simulink model "ExoTeR"  (R2019b)
settings: Solver=VariableStepAuto  StartTime=0.0  StopTime=t(end)  MaxStep=0.001  RelTol=1e-6  AbsTol=1e-6  EnableMultiTasking=on
undefined symbols (not defined in the file): a2, a3, d1, d4, d5, d6, g, Housing, ki, kp, l, m1, m2, m3, m4, m5, mu, q, rollef, s, slope, theta, vehicleMass, wheelMass, wheelRadius, x, X, xef, Y, yef, Z, zGC
libraries: sm_lib x187, fl_lib x99, nesl_utility x45, ee_lib x12, simulink x6
(part 6 of 7)

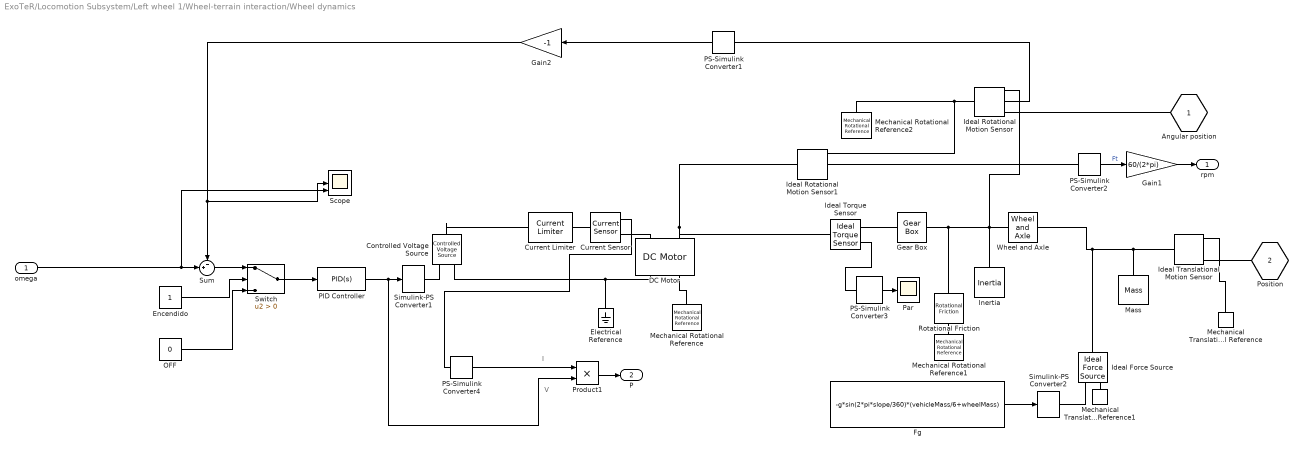
== system ExoTeR/Locomotion Subsystem/Left wheel 1/Wheel-terrain interaction/Wheel dynamics ==
  note: V
  note: I
  omega : Inport
  Controlled Voltage Source : fl_lib/Electrical/Electrical Sources/Controlled Voltage Source
  Current Limiter : ee_lib/Semiconductors & Converters/Current Limiter  iLim=0.5 A  vLim=0.01 V  gLim=1e-3 1/Ohm  thermal_mass=100 J/K  initial_temperature=298.15 K
      settings: SourceProductName=Simscape Electrical  SourceProductBaseCode=PS  InternalSimscapePortConfiguration="{\"Bottom\":[],\"Left\":[{\"id\":\"p\",\"label\":\"+\",\"type\":\"foundation.electrical.electrical\"}],\"Right\":[{\"id\":\"n\",\"label\":\"-\",\"type\":\"foundation.electrical.electrical\"}],\"Top\":[]}"
  Current Sensor : fl_lib/Electrical/Electrical Sensors/Current Sensor
  DC Motor : ee_lib/Electromechanical/Brushed Motors/DC Motor  parameterization=2  Ra=3.9 Ohm  La=0.000363 H  emf_or_torque=2  Kv=0.0011 V/rpm  Ki=10.9 mN*m/A  T_stall=0.0237 N*m  w_max=10200 rpm  w_rated=1.5e+4 rpm  P_rated=0.08 W  V_rated=12 V  J=4.36 g*cm^2  lam_param=2  lam=Bm N*m/(rad/s)  i_noload=0.0458 A  V_i_noload=11.657 V  speed0=0 rpm  alpha=3.93e-3 1/K  Tmeas=25 degC  thermal_mass=100 J/K  initial_temperature=25 degC
      settings: SourceProductName=Simscape Electrical
  Electrical Reference : fl_lib/Electrical/Electrical Elements/Electrical Reference
  Encendido : Constant
  Fg : Constant  Value=-g*sin(2*pi*slope/360)*(vehicleMass/6+wheelMass)
  Gain1 : Gain  Gain=60/(2*pi)
  Gain2 : Gain  Gain=-1
  Gear Box : fl_lib/Mechanical/Mechanisms/Gear Box  ratio=675.545  t_in_specify=off  t_in_priority=None  t_in=0 N*m  t_in_nominal_specify=off  t_in_nominal_unit=N*m  t_in_nominal_value=1  t_out_specify=off  t_out_priority=None  t_out=0 N*m  t_out_nominal_specify=off  t_out_nominal_unit=N*m  t_out_nominal_value=1
  Ideal Force Source : fl_lib/Mechanical/Mechanical Sources/Ideal Force Source
  Ideal Rotational Motion Sensor : fl_lib/Mechanical/Mechanical Sensors/Ideal Rotational Motion Sensor  offset=0 rad
  Ideal Rotational Motion Sensor1 : fl_lib/Mechanical/Mechanical Sensors/Ideal Rotational Motion Sensor  offset=0 rad
  Ideal Torque Sensor : fl_lib/Mechanical/Mechanical Sensors/Ideal Torque Sensor
  Ideal Translational Motion Sensor : fl_lib/Mechanical/Mechanical Sensors/Ideal Translational Motion Sensor  offset=0 m
  Inertia : fl_lib/Mechanical/Rotational Elements/Inertia  inertia=Jw kg*m^2  w_specify=off  w_priority=None  w=0 rad/s  w_nominal_specify=off  w_nominal_unit=rad/s  w_nominal_value=1  t_specify=off  t_priority=None  t=0 N*m  t_nominal_specify=off  t_nominal_unit=N*m  t_nominal_value=1
  Mass : fl_lib/Mechanical/Translational Elements/Mass  mass=vehicleMass/6+wheelMass kg  v_specify=off  v_priority=None  v=0 m/s  v_nominal_specify=off  v_nominal_unit=m/s  v_nominal_value=1  f_specify=off  f_priority=None  f=0 N  f_nominal_specify=off  f_nominal_unit=N  f_nominal_value=1
  Mechanical Rotational Reference : fl_lib/Mechanical/Rotational Elements/Mechanical Rotational Reference
  Mechanical Rotational Reference1 : fl_lib/Mechanical/Rotational Elements/Mechanical Rotational Reference
  Mechanical Rotational Reference2 : fl_lib/Mechanical/Rotational Elements/Mechanical Rotational Reference
  Mechanical Translational Reference : fl_lib/Mechanical/Translational Elements/Mechanical Translational Reference
  Mechanical Translational Reference1 : fl_lib/Mechanical/Translational Elements/Mechanical Translational Reference
  OFF : Constant  Value=0
  PID Controller : simulink/Continuous/PID Controller  Controller=PID  Form=Parallel  TimeDomain=Continuous-time  SampleTime=-1  IntegratorMethod=Forward Euler  FilterMethod=Forward Euler  ControllerParametersSource=internal  P=kp  I=ki  D=0  UseFilter=on  N=100  TunerSelectOption=Transfer Function Based (PID Tuner App)  InitialConditionSource=internal  InitialConditionForIntegrator=0  InitialConditionForFilter=0  DifferentiatorICPrevScaledInput=0  ExternalReset=none  TrackingMode=off  Kt=1  LimitOutput=on  UpperSaturationLimit=12  LowerSaturationLimit=-12  LinearizeAsGain=on  AntiWindupMode=back-calculation  Kb=1  POutMin=[]  POutMax=[]  IOutMin=[]  IOutMax=[]  DOutMin=[]  DOutMax=[]  NOutMin=[]  NOutMax=[]  SumOutMin=[]  SumOutMax=[]  SaturationOutMin=[]  SaturationOutMax=[]  PParamMin=[]  PParamMax=[]  IParamMin=[]  IParamMax=[]  DParamMin=[]  DParamMax=[]  NParamMin=[]  NParamMax=[]  KbParamMin=[]  KbParamMax=[]  KtParamMin=[]  KtParamMax=[]  KbOutMin=[]  KbOutMax=[]  KtOutMin=[]  KtOutMax=[]  IntegratorOutMin=[]  IntegratorOutMax=[]  FilterOutMin=[]  FilterOutMax=[]  SumI1OutMin=[]  SumI1OutMax=[]  SumI2OutMin=[]  SumI2OutMax=[]  SumI3OutMin=[]  SumI3OutMax=[]  SumI4OutMin=[]  SumI4OutMax=[]  SumDOutMin=[]  SumDOutMax=[]  DifferentiatorOutMin=[]  DifferentiatorOutMax=[]  FilterDiffOutCoefMin=[]  FilterDiffOutCoefMax=[]  ReciprocalOutMin=[]  ReciprocalOutMax=[]  SumDenOutMin=[]  SumDenOutMax=[]  SumNumOutMin=[]  SumNumOutMax=[]  DivideOutMin=[]  DivideOutMax=[]  IntegratorContinuousStateAttributes=''  IntegratorStateMustResolveToSignalObject=off  IntegratorRTWStateStorageClass=Auto  FilterContinuousStateAttributes=''  FilterStateMustResolveToSignalObject=off  FilterRTWStateStorageClass=Auto  ParallelPVariant=InternalParameters  IdealPVariant=Disabled  IVariant=InternalParameters  DVariant=InternalParameters  IntegratorVariant=Continuous  SatVariant=Enabled  AWVariant=BackCalculation  PCopyVariant=Disabled  TRVariant=Disabled  FdbkBlocksVariant=Forward  IdealPFdbkVariant=Disabled  SatFdbkVariant=Disabled  DerivativeFilterVariant=ContFilter  NVariant=InternalParameters  NCopyVariant=Disabled  FilterICVariant=InternalICsFilter  IntegratorICVariant=InternalICs  ExternalResetVariant=Disabled  TRSumVariant=Passthrough  SumFdbkVariant=Disabled  SumVariant=Sum_PID
  PS-Simulink Converter{1..4} (4 alike) : nesl_utility/PS-Simulink Converter  PhysicalDomain=network_engine_domain  SubClassName=ps_output  LeftPortType=input  RightPortType=output  PseudoPeriodic=off  Frequencies=[]  Unit=1  AffineConversion=off
  Par : Scope
  Product1 : Product
  Rotational Friction : fl_lib/Mechanical/Rotational Elements/Rotational Friction  brkwy_trq=(vehicleMass/6+wheelMass)*g*cos(2*pi*slope/360)*mu*wheelRadius*s + (vehicleMass/6+wheelMass)*g*cos(2*pi*slope/360)*mu*0.1*wheelRadius*(1-s) N*m  brkwy_vel=0.060623 rad/s  Col_trq=((vehicleMass/6+wheelMass)*g*cos(2*pi*slope/360)*mu*wheelRadius*s + (vehicleMass/6+wheelMass)*g*cos(2*pi*slope/360)*mu*0.1*wheelRadius*(1-s))*0.9 N*m  visc_coef=0.001 N*m/(rad/s)  w_specify=off  w_priority=None  w=0 rad/s  w_nominal_specify=off  w_nominal_unit=rad/s  w_nominal_value=1  t_specify=off  t_priority=None  t=0 N*m  t_nominal_specify=off  t_nominal_unit=N*m  t_nominal_value=1
      settings: SourceProductName=Simscape
  Scope : Scope  NumInputPorts=3
  Simulink-PS Converter1 : nesl_utility/Simulink-PS Converter  PhysicalDomain=network_engine_domain  SubClassName=ps_input  LeftPortType=input  RightPortType=output  PseudoPeriodic=off  Frequencies=[]  NoiseDistribution=none  NoiseParameters=[]  Unit=1  AffineConversion=off  FilteringAndDerivatives=zero  SimscapeFilterOrder=1  InputFilterTimeConstant=0.001  UdotUserProvided=1
  Simulink-PS Converter2 : nesl_utility/Simulink-PS Converter  PhysicalDomain=network_engine_domain  SubClassName=ps_input  LeftPortType=input  RightPortType=output  PseudoPeriodic=off  Frequencies=[]  NoiseDistribution=none  NoiseParameters=[]  Unit=1  AffineConversion=off  FilteringAndDerivatives=zero  SimscapeFilterOrder=1  InputFilterTimeConstant=0.001  UdotUserProvided=1
  Sum : Sum  Inputs=-+|
  Switch : Switch  Criteria=u2 > Threshold
  Wheel and Axle : fl_lib/Mechanical/Mechanisms/Wheel and Axle  R=wheelRadius m  or=1  t_specify=off  t_priority=None  t=0 N*m  t_nominal_specify=off  t_nominal_unit=N*m  t_nominal_value=1  f_specify=off  f_priority=None  f=0 N  f_nominal_specify=off  f_nominal_unit=N  f_nominal_value=1
      settings: SourceProductName=Simscape
  Angular position : PMIOPort  Side=Right
  Position : PMIOPort  Port=2  Side=Right
  rpm : Outport
  P : Outport  Port=2
  wires:
  PS-Simulink Converter2/1 -> Gain1/1  "Ft"
  Gain1/1 -> rpm/1
  Fg/1 -> Simulink-PS Converter2/1
  PID Controller/1 -> Product1/2, Simulink-PS Converter1/1
  PS-Simulink Converter1/1 -> Gain2/1
  omega/1 -> Scope/3, Sum/2
  Gain2/1 -> Scope/2, Sum/1
  Encendido/1 -> Switch/2
  OFF/1 -> Switch/3
  Switch/1 -> PID Controller/1
  Sum/1 -> Switch/1
  PS-Simulink Converter3/1 -> Par/1
  PS-Simulink Converter4/1 -> Product1/1
  Product1/1 -> P/1
  connections:
  Inertia/LConn1 -- Rotational Friction/LConn1 -- Gear Box/RConn1 -- Ideal Rotational Motion Sensor/RConn1 -- Wheel and Axle/LConn1
  DC Motor/RConn2 -- Mechanical Rotational Reference/LConn1
  Ideal Rotational Motion Sensor1/LConn1 -- Ideal Torque Sensor/LConn1 -- DC Motor/LConn2
  Mechanical Translational Reference/LConn1 -- Ideal Translational Motion Sensor/RConn1
  Electrical Reference/LConn1 -- DC Motor/RConn1 -- Controlled Voltage Source/RConn2
  Simulink-PS Converter1/RConn1 -- Controlled Voltage Source/RConn1
  Mechanical Rotational Reference1/LConn1 -- Rotational Friction/RConn1
  Ideal Rotational Motion Sensor/RConn3 -- Angular position/RConn1
  Ideal Translational Motion Sensor/RConn3 -- Position/RConn1
  Mechanical Rotational Reference2/LConn1 -- Ideal Rotational Motion Sensor1/RConn1 -- Ideal Rotational Motion Sensor/LConn1
  Ideal Rotational Motion Sensor1/RConn2 -- PS-Simulink Converter2/LConn1
  Simulink-PS Converter2/RConn1 -- Ideal Force Source/RConn1
  Mechanical Translational Reference1/LConn1 -- Ideal Force Source/RConn2
  Ideal Translational Motion Sensor/LConn1 -- Wheel and Axle/RConn1 -- Ideal Force Source/LConn1 -- Mass/LConn1
  Ideal Rotational Motion Sensor/RConn2 -- PS-Simulink Converter1/LConn1
  Ideal Torque Sensor/RConn1 -- Gear Box/LConn1
  Ideal Torque Sensor/RConn2 -- PS-Simulink Converter3/LConn1
  Controlled Voltage Source/LConn1 -- Current Limiter/LConn1
  Current Sensor/RConn1 -- PS-Simulink Converter4/LConn1
  Current Limiter/RConn1 -- Current Sensor/LConn1
  Current Sensor/RConn2 -- DC Motor/LConn1

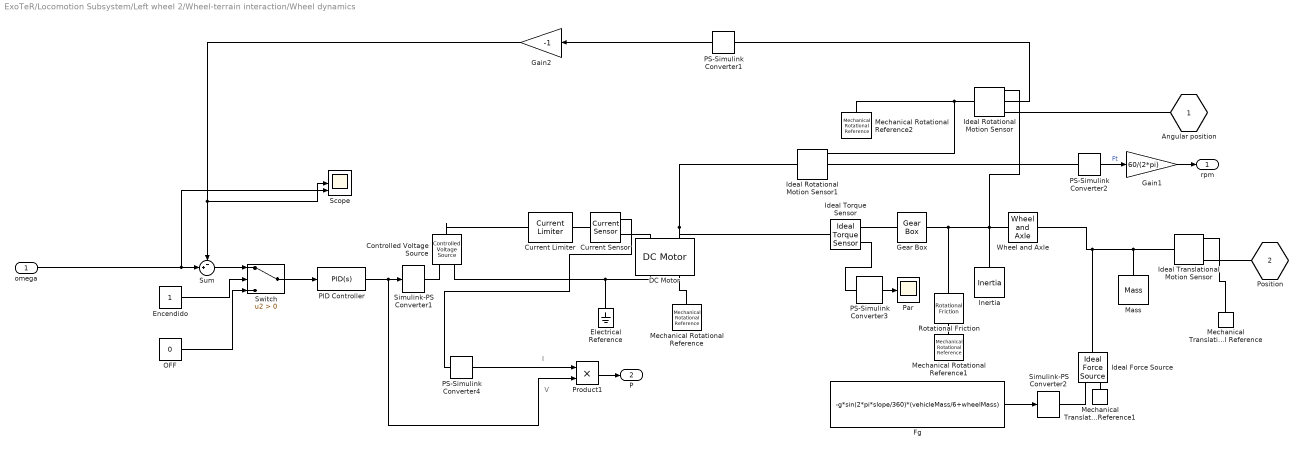
== system ExoTeR/Locomotion Subsystem/Left wheel 2/Wheel-terrain interaction/Wheel dynamics ==
  note: V
  note: I
  omega : Inport
  Controlled Voltage Source : fl_lib/Electrical/Electrical Sources/Controlled Voltage Source
  Current Limiter : ee_lib/Semiconductors & Converters/Current Limiter  iLim=0.5 A  vLim=0.01 V  gLim=1e-3 1/Ohm  thermal_mass=100 J/K  initial_temperature=298.15 K
      settings: SourceProductName=Simscape Electrical  SourceProductBaseCode=PS  InternalSimscapePortConfiguration="{\"Bottom\":[],\"Left\":[{\"id\":\"p\",\"label\":\"+\",\"type\":\"foundation.electrical.electrical\"}],\"Right\":[{\"id\":\"n\",\"label\":\"-\",\"type\":\"foundation.electrical.electrical\"}],\"Top\":[]}"
  Current Sensor : fl_lib/Electrical/Electrical Sensors/Current Sensor
  DC Motor : ee_lib/Electromechanical/Brushed Motors/DC Motor  parameterization=2  Ra=3.9 Ohm  La=0.000363 H  emf_or_torque=2  Kv=0.0011 V/rpm  Ki=10.9 mN*m/A  T_stall=0.0237 N*m  w_max=10200 rpm  w_rated=1.5e+4 rpm  P_rated=0.08 W  V_rated=12 V  J=4.36 g*cm^2  lam_param=2  lam=Bm N*m/(rad/s)  i_noload=0.0458 A  V_i_noload=11.657 V  speed0=0 rpm  alpha=3.93e-3 1/K  Tmeas=25 degC  thermal_mass=100 J/K  initial_temperature=25 degC
      settings: SourceProductName=Simscape Electrical
  Electrical Reference : fl_lib/Electrical/Electrical Elements/Electrical Reference
  Encendido : Constant
  Fg : Constant  Value=-g*sin(2*pi*slope/360)*(vehicleMass/6+wheelMass)
  Gain1 : Gain  Gain=60/(2*pi)
  Gain2 : Gain  Gain=-1
  Gear Box : fl_lib/Mechanical/Mechanisms/Gear Box  ratio=675.545  t_in_specify=off  t_in_priority=None  t_in=0 N*m  t_in_nominal_specify=off  t_in_nominal_unit=N*m  t_in_nominal_value=1  t_out_specify=off  t_out_priority=None  t_out=0 N*m  t_out_nominal_specify=off  t_out_nominal_unit=N*m  t_out_nominal_value=1
  Ideal Force Source : fl_lib/Mechanical/Mechanical Sources/Ideal Force Source
  Ideal Rotational Motion Sensor : fl_lib/Mechanical/Mechanical Sensors/Ideal Rotational Motion Sensor  offset=0 rad
  Ideal Rotational Motion Sensor1 : fl_lib/Mechanical/Mechanical Sensors/Ideal Rotational Motion Sensor  offset=0 rad
  Ideal Torque Sensor : fl_lib/Mechanical/Mechanical Sensors/Ideal Torque Sensor
  Ideal Translational Motion Sensor : fl_lib/Mechanical/Mechanical Sensors/Ideal Translational Motion Sensor  offset=0 m
  Inertia : fl_lib/Mechanical/Rotational Elements/Inertia  inertia=Jw kg*m^2  w_specify=off  w_priority=None  w=0 rad/s  w_nominal_specify=off  w_nominal_unit=rad/s  w_nominal_value=1  t_specify=off  t_priority=None  t=0 N*m  t_nominal_specify=off  t_nominal_unit=N*m  t_nominal_value=1
  Mass : fl_lib/Mechanical/Translational Elements/Mass  mass=vehicleMass/6+wheelMass kg  v_specify=off  v_priority=None  v=0 m/s  v_nominal_specify=off  v_nominal_unit=m/s  v_nominal_value=1  f_specify=off  f_priority=None  f=0 N  f_nominal_specify=off  f_nominal_unit=N  f_nominal_value=1
  Mechanical Rotational Reference : fl_lib/Mechanical/Rotational Elements/Mechanical Rotational Reference
  Mechanical Rotational Reference1 : fl_lib/Mechanical/Rotational Elements/Mechanical Rotational Reference
  Mechanical Rotational Reference2 : fl_lib/Mechanical/Rotational Elements/Mechanical Rotational Reference
  Mechanical Translational Reference : fl_lib/Mechanical/Translational Elements/Mechanical Translational Reference
  Mechanical Translational Reference1 : fl_lib/Mechanical/Translational Elements/Mechanical Translational Reference
  OFF : Constant  Value=0
  PID Controller : simulink/Continuous/PID Controller  Controller=PID  Form=Parallel  TimeDomain=Continuous-time  SampleTime=-1  IntegratorMethod=Forward Euler  FilterMethod=Forward Euler  ControllerParametersSource=internal  P=kp  I=ki  D=0  UseFilter=on  N=100  TunerSelectOption=Transfer Function Based (PID Tuner App)  InitialConditionSource=internal  InitialConditionForIntegrator=0  InitialConditionForFilter=0  DifferentiatorICPrevScaledInput=0  ExternalReset=none  TrackingMode=off  Kt=1  LimitOutput=on  UpperSaturationLimit=12  LowerSaturationLimit=-12  LinearizeAsGain=on  AntiWindupMode=back-calculation  Kb=1  POutMin=[]  POutMax=[]  IOutMin=[]  IOutMax=[]  DOutMin=[]  DOutMax=[]  NOutMin=[]  NOutMax=[]  SumOutMin=[]  SumOutMax=[]  SaturationOutMin=[]  SaturationOutMax=[]  PParamMin=[]  PParamMax=[]  IParamMin=[]  IParamMax=[]  DParamMin=[]  DParamMax=[]  NParamMin=[]  NParamMax=[]  KbParamMin=[]  KbParamMax=[]  KtParamMin=[]  KtParamMax=[]  KbOutMin=[]  KbOutMax=[]  KtOutMin=[]  KtOutMax=[]  IntegratorOutMin=[]  IntegratorOutMax=[]  FilterOutMin=[]  FilterOutMax=[]  SumI1OutMin=[]  SumI1OutMax=[]  SumI2OutMin=[]  SumI2OutMax=[]  SumI3OutMin=[]  SumI3OutMax=[]  SumI4OutMin=[]  SumI4OutMax=[]  SumDOutMin=[]  SumDOutMax=[]  DifferentiatorOutMin=[]  DifferentiatorOutMax=[]  FilterDiffOutCoefMin=[]  FilterDiffOutCoefMax=[]  ReciprocalOutMin=[]  ReciprocalOutMax=[]  SumDenOutMin=[]  SumDenOutMax=[]  SumNumOutMin=[]  SumNumOutMax=[]  DivideOutMin=[]  DivideOutMax=[]  IntegratorContinuousStateAttributes=''  IntegratorStateMustResolveToSignalObject=off  IntegratorRTWStateStorageClass=Auto  FilterContinuousStateAttributes=''  FilterStateMustResolveToSignalObject=off  FilterRTWStateStorageClass=Auto  ParallelPVariant=InternalParameters  IdealPVariant=Disabled  IVariant=InternalParameters  DVariant=InternalParameters  IntegratorVariant=Continuous  SatVariant=Enabled  AWVariant=BackCalculation  PCopyVariant=Disabled  TRVariant=Disabled  FdbkBlocksVariant=Forward  IdealPFdbkVariant=Disabled  SatFdbkVariant=Disabled  DerivativeFilterVariant=ContFilter  NVariant=InternalParameters  NCopyVariant=Disabled  FilterICVariant=InternalICsFilter  IntegratorICVariant=InternalICs  ExternalResetVariant=Disabled  TRSumVariant=Passthrough  SumFdbkVariant=Disabled  SumVariant=Sum_PID
  PS-Simulink Converter{1..4} (4 alike) : nesl_utility/PS-Simulink Converter  PhysicalDomain=network_engine_domain  SubClassName=ps_output  LeftPortType=input  RightPortType=output  PseudoPeriodic=off  Frequencies=[]  Unit=1  AffineConversion=off
  Par : Scope
  Product1 : Product
  Rotational Friction : fl_lib/Mechanical/Rotational Elements/Rotational Friction  brkwy_trq=(vehicleMass/6+wheelMass)*g*cos(2*pi*slope/360)*mu*wheelRadius*s + (vehicleMass/6+wheelMass)*g*cos(2*pi*slope/360)*mu*0.1*wheelRadius*(1-s) N*m  brkwy_vel=0.060623 rad/s  Col_trq=((vehicleMass/6+wheelMass)*g*cos(2*pi*slope/360)*mu*wheelRadius*s + (vehicleMass/6+wheelMass)*g*cos(2*pi*slope/360)*mu*0.1*wheelRadius*(1-s))*0.9 N*m  visc_coef=0.001 N*m/(rad/s)  w_specify=off  w_priority=None  w=0 rad/s  w_nominal_specify=off  w_nominal_unit=rad/s  w_nominal_value=1  t_specify=off  t_priority=None  t=0 N*m  t_nominal_specify=off  t_nominal_unit=N*m  t_nominal_value=1
      settings: SourceProductName=Simscape
  Scope : Scope  NumInputPorts=3
  Simulink-PS Converter1 : nesl_utility/Simulink-PS Converter  PhysicalDomain=network_engine_domain  SubClassName=ps_input  LeftPortType=input  RightPortType=output  PseudoPeriodic=off  Frequencies=[]  NoiseDistribution=none  NoiseParameters=[]  Unit=1  AffineConversion=off  FilteringAndDerivatives=zero  SimscapeFilterOrder=1  InputFilterTimeConstant=0.001  UdotUserProvided=1
  Simulink-PS Converter2 : nesl_utility/Simulink-PS Converter  PhysicalDomain=network_engine_domain  SubClassName=ps_input  LeftPortType=input  RightPortType=output  PseudoPeriodic=off  Frequencies=[]  NoiseDistribution=none  NoiseParameters=[]  Unit=1  AffineConversion=off  FilteringAndDerivatives=zero  SimscapeFilterOrder=1  InputFilterTimeConstant=0.001  UdotUserProvided=1
  Sum : Sum  Inputs=-+|
  Switch : Switch  Criteria=u2 > Threshold
  Wheel and Axle : fl_lib/Mechanical/Mechanisms/Wheel and Axle  R=wheelRadius m  or=1  t_specify=off  t_priority=None  t=0 N*m  t_nominal_specify=off  t_nominal_unit=N*m  t_nominal_value=1  f_specify=off  f_priority=None  f=0 N  f_nominal_specify=off  f_nominal_unit=N  f_nominal_value=1
      settings: SourceProductName=Simscape
  Angular position : PMIOPort  Side=Right
  Position : PMIOPort  Port=2  Side=Right
  rpm : Outport
  P : Outport  Port=2
  wires:
  PS-Simulink Converter2/1 -> Gain1/1  "Ft"
  Gain1/1 -> rpm/1
  Fg/1 -> Simulink-PS Converter2/1
  PID Controller/1 -> Product1/2, Simulink-PS Converter1/1
  PS-Simulink Converter1/1 -> Gain2/1
  omega/1 -> Scope/3, Sum/2
  Gain2/1 -> Scope/2, Sum/1
  Encendido/1 -> Switch/2
  OFF/1 -> Switch/3
  Switch/1 -> PID Controller/1
  Sum/1 -> Switch/1
  PS-Simulink Converter3/1 -> Par/1
  PS-Simulink Converter4/1 -> Product1/1
  Product1/1 -> P/1
  connections:
  Inertia/LConn1 -- Rotational Friction/LConn1 -- Gear Box/RConn1 -- Ideal Rotational Motion Sensor/RConn1 -- Wheel and Axle/LConn1
  DC Motor/RConn2 -- Mechanical Rotational Reference/LConn1
  Ideal Rotational Motion Sensor1/LConn1 -- Ideal Torque Sensor/LConn1 -- DC Motor/LConn2
  Mechanical Translational Reference/LConn1 -- Ideal Translational Motion Sensor/RConn1
  Electrical Reference/LConn1 -- DC Motor/RConn1 -- Controlled Voltage Source/RConn2
  Simulink-PS Converter1/RConn1 -- Controlled Voltage Source/RConn1
  Mechanical Rotational Reference1/LConn1 -- Rotational Friction/RConn1
  Ideal Rotational Motion Sensor/RConn3 -- Angular position/RConn1
  Ideal Translational Motion Sensor/RConn3 -- Position/RConn1
  Mechanical Rotational Reference2/LConn1 -- Ideal Rotational Motion Sensor1/RConn1 -- Ideal Rotational Motion Sensor/LConn1
  Ideal Rotational Motion Sensor1/RConn2 -- PS-Simulink Converter2/LConn1
  Simulink-PS Converter2/RConn1 -- Ideal Force Source/RConn1
  Mechanical Translational Reference1/LConn1 -- Ideal Force Source/RConn2
  Ideal Translational Motion Sensor/LConn1 -- Wheel and Axle/RConn1 -- Ideal Force Source/LConn1 -- Mass/LConn1
  Ideal Rotational Motion Sensor/RConn2 -- PS-Simulink Converter1/LConn1
  Ideal Torque Sensor/RConn1 -- Gear Box/LConn1
  Ideal Torque Sensor/RConn2 -- PS-Simulink Converter3/LConn1
  Controlled Voltage Source/LConn1 -- Current Limiter/LConn1
  Current Sensor/RConn1 -- PS-Simulink Converter4/LConn1
  Current Limiter/RConn1 -- Current Sensor/LConn1
  Current Sensor/RConn2 -- DC Motor/LConn1

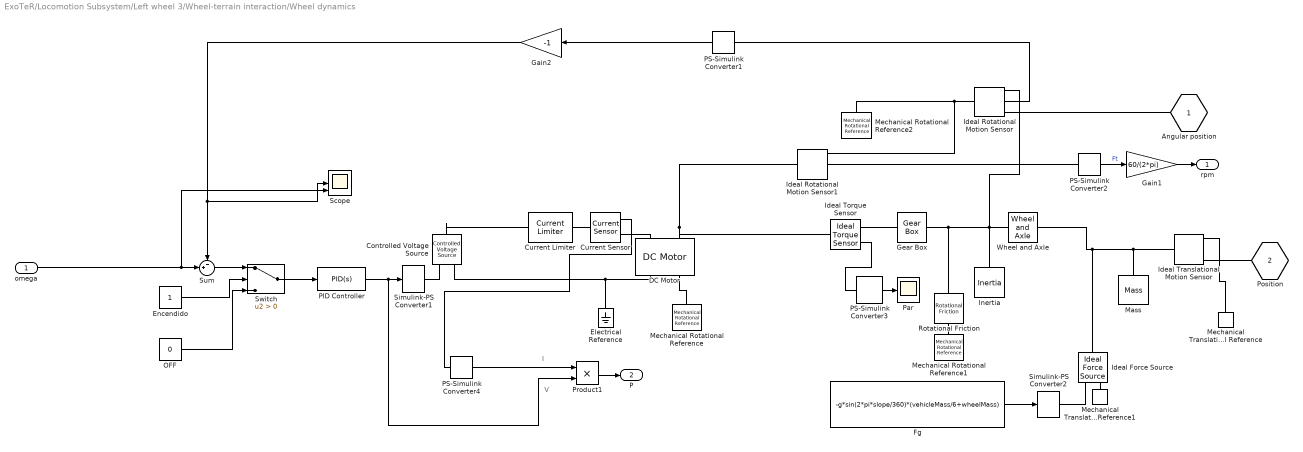
== system ExoTeR/Locomotion Subsystem/Left wheel 3/Wheel-terrain interaction/Wheel dynamics ==
  note: V
  note: I
  omega : Inport
  Controlled Voltage Source : fl_lib/Electrical/Electrical Sources/Controlled Voltage Source
  Current Limiter : ee_lib/Semiconductors & Converters/Current Limiter  iLim=0.5 A  vLim=0.01 V  gLim=1e-3 1/Ohm  thermal_mass=100 J/K  initial_temperature=298.15 K
      settings: SourceProductName=Simscape Electrical  SourceProductBaseCode=PS  InternalSimscapePortConfiguration="{\"Bottom\":[],\"Left\":[{\"id\":\"p\",\"label\":\"+\",\"type\":\"foundation.electrical.electrical\"}],\"Right\":[{\"id\":\"n\",\"label\":\"-\",\"type\":\"foundation.electrical.electrical\"}],\"Top\":[]}"
  Current Sensor : fl_lib/Electrical/Electrical Sensors/Current Sensor
  DC Motor : ee_lib/Electromechanical/Brushed Motors/DC Motor  parameterization=2  Ra=3.9 Ohm  La=0.000363 H  emf_or_torque=2  Kv=0.0011 V/rpm  Ki=10.9 mN*m/A  T_stall=0.0237 N*m  w_max=10200 rpm  w_rated=1.5e+4 rpm  P_rated=0.08 W  V_rated=12 V  J=4.36 g*cm^2  lam_param=2  lam=Bm N*m/(rad/s)  i_noload=0.0458 A  V_i_noload=11.657 V  speed0=0 rpm  alpha=3.93e-3 1/K  Tmeas=25 degC  thermal_mass=100 J/K  initial_temperature=25 degC
      settings: SourceProductName=Simscape Electrical
  Electrical Reference : fl_lib/Electrical/Electrical Elements/Electrical Reference
  Encendido : Constant
  Fg : Constant  Value=-g*sin(2*pi*slope/360)*(vehicleMass/6+wheelMass)
  Gain1 : Gain  Gain=60/(2*pi)
  Gain2 : Gain  Gain=-1
  Gear Box : fl_lib/Mechanical/Mechanisms/Gear Box  ratio=675.545  t_in_specify=off  t_in_priority=None  t_in=0 N*m  t_in_nominal_specify=off  t_in_nominal_unit=N*m  t_in_nominal_value=1  t_out_specify=off  t_out_priority=None  t_out=0 N*m  t_out_nominal_specify=off  t_out_nominal_unit=N*m  t_out_nominal_value=1
  Ideal Force Source : fl_lib/Mechanical/Mechanical Sources/Ideal Force Source
  Ideal Rotational Motion Sensor : fl_lib/Mechanical/Mechanical Sensors/Ideal Rotational Motion Sensor  offset=0 rad
  Ideal Rotational Motion Sensor1 : fl_lib/Mechanical/Mechanical Sensors/Ideal Rotational Motion Sensor  offset=0 rad
  Ideal Torque Sensor : fl_lib/Mechanical/Mechanical Sensors/Ideal Torque Sensor
  Ideal Translational Motion Sensor : fl_lib/Mechanical/Mechanical Sensors/Ideal Translational Motion Sensor  offset=0 m
  Inertia : fl_lib/Mechanical/Rotational Elements/Inertia  inertia=Jw kg*m^2  w_specify=off  w_priority=None  w=0 rad/s  w_nominal_specify=off  w_nominal_unit=rad/s  w_nominal_value=1  t_specify=off  t_priority=None  t=0 N*m  t_nominal_specify=off  t_nominal_unit=N*m  t_nominal_value=1
  Mass : fl_lib/Mechanical/Translational Elements/Mass  mass=vehicleMass/6+wheelMass kg  v_specify=off  v_priority=None  v=0 m/s  v_nominal_specify=off  v_nominal_unit=m/s  v_nominal_value=1  f_specify=off  f_priority=None  f=0 N  f_nominal_specify=off  f_nominal_unit=N  f_nominal_value=1
  Mechanical Rotational Reference : fl_lib/Mechanical/Rotational Elements/Mechanical Rotational Reference
  Mechanical Rotational Reference1 : fl_lib/Mechanical/Rotational Elements/Mechanical Rotational Reference
  Mechanical Rotational Reference2 : fl_lib/Mechanical/Rotational Elements/Mechanical Rotational Reference
  Mechanical Translational Reference : fl_lib/Mechanical/Translational Elements/Mechanical Translational Reference
  Mechanical Translational Reference1 : fl_lib/Mechanical/Translational Elements/Mechanical Translational Reference
  OFF : Constant  Value=0
  PID Controller : simulink/Continuous/PID Controller  Controller=PID  Form=Parallel  TimeDomain=Continuous-time  SampleTime=-1  IntegratorMethod=Forward Euler  FilterMethod=Forward Euler  ControllerParametersSource=internal  P=kp  I=ki  D=0  UseFilter=on  N=100  TunerSelectOption=Transfer Function Based (PID Tuner App)  InitialConditionSource=internal  InitialConditionForIntegrator=0  InitialConditionForFilter=0  DifferentiatorICPrevScaledInput=0  ExternalReset=none  TrackingMode=off  Kt=1  LimitOutput=on  UpperSaturationLimit=12  LowerSaturationLimit=-12  LinearizeAsGain=on  AntiWindupMode=back-calculation  Kb=1  POutMin=[]  POutMax=[]  IOutMin=[]  IOutMax=[]  DOutMin=[]  DOutMax=[]  NOutMin=[]  NOutMax=[]  SumOutMin=[]  SumOutMax=[]  SaturationOutMin=[]  SaturationOutMax=[]  PParamMin=[]  PParamMax=[]  IParamMin=[]  IParamMax=[]  DParamMin=[]  DParamMax=[]  NParamMin=[]  NParamMax=[]  KbParamMin=[]  KbParamMax=[]  KtParamMin=[]  KtParamMax=[]  KbOutMin=[]  KbOutMax=[]  KtOutMin=[]  KtOutMax=[]  IntegratorOutMin=[]  IntegratorOutMax=[]  FilterOutMin=[]  FilterOutMax=[]  SumI1OutMin=[]  SumI1OutMax=[]  SumI2OutMin=[]  SumI2OutMax=[]  SumI3OutMin=[]  SumI3OutMax=[]  SumI4OutMin=[]  SumI4OutMax=[]  SumDOutMin=[]  SumDOutMax=[]  DifferentiatorOutMin=[]  DifferentiatorOutMax=[]  FilterDiffOutCoefMin=[]  FilterDiffOutCoefMax=[]  ReciprocalOutMin=[]  ReciprocalOutMax=[]  SumDenOutMin=[]  SumDenOutMax=[]  SumNumOutMin=[]  SumNumOutMax=[]  DivideOutMin=[]  DivideOutMax=[]  IntegratorContinuousStateAttributes=''  IntegratorStateMustResolveToSignalObject=off  IntegratorRTWStateStorageClass=Auto  FilterContinuousStateAttributes=''  FilterStateMustResolveToSignalObject=off  FilterRTWStateStorageClass=Auto  ParallelPVariant=InternalParameters  IdealPVariant=Disabled  IVariant=InternalParameters  DVariant=InternalParameters  IntegratorVariant=Continuous  SatVariant=Enabled  AWVariant=BackCalculation  PCopyVariant=Disabled  TRVariant=Disabled  FdbkBlocksVariant=Forward  IdealPFdbkVariant=Disabled  SatFdbkVariant=Disabled  DerivativeFilterVariant=ContFilter  NVariant=InternalParameters  NCopyVariant=Disabled  FilterICVariant=InternalICsFilter  IntegratorICVariant=InternalICs  ExternalResetVariant=Disabled  TRSumVariant=Passthrough  SumFdbkVariant=Disabled  SumVariant=Sum_PID
  PS-Simulink Converter{1..4} (4 alike) : nesl_utility/PS-Simulink Converter  PhysicalDomain=network_engine_domain  SubClassName=ps_output  LeftPortType=input  RightPortType=output  PseudoPeriodic=off  Frequencies=[]  Unit=1  AffineConversion=off
  Par : Scope
  Product1 : Product
  Rotational Friction : fl_lib/Mechanical/Rotational Elements/Rotational Friction  brkwy_trq=(vehicleMass/6+wheelMass)*g*cos(2*pi*slope/360)*mu*wheelRadius*s + (vehicleMass/6+wheelMass)*g*cos(2*pi*slope/360)*mu*0.1*wheelRadius*(1-s) N*m  brkwy_vel=0.060623 rad/s  Col_trq=((vehicleMass/6+wheelMass)*g*cos(2*pi*slope/360)*mu*wheelRadius*s + (vehicleMass/6+wheelMass)*g*cos(2*pi*slope/360)*mu*0.1*wheelRadius*(1-s))*0.9 N*m  visc_coef=0.001 N*m/(rad/s)  w_specify=off  w_priority=None  w=0 rad/s  w_nominal_specify=off  w_nominal_unit=rad/s  w_nominal_value=1  t_specify=off  t_priority=None  t=0 N*m  t_nominal_specify=off  t_nominal_unit=N*m  t_nominal_value=1
      settings: SourceProductName=Simscape
  Scope : Scope  NumInputPorts=3
  Simulink-PS Converter1 : nesl_utility/Simulink-PS Converter  PhysicalDomain=network_engine_domain  SubClassName=ps_input  LeftPortType=input  RightPortType=output  PseudoPeriodic=off  Frequencies=[]  NoiseDistribution=none  NoiseParameters=[]  Unit=1  AffineConversion=off  FilteringAndDerivatives=zero  SimscapeFilterOrder=1  InputFilterTimeConstant=0.001  UdotUserProvided=1
  Simulink-PS Converter2 : nesl_utility/Simulink-PS Converter  PhysicalDomain=network_engine_domain  SubClassName=ps_input  LeftPortType=input  RightPortType=output  PseudoPeriodic=off  Frequencies=[]  NoiseDistribution=none  NoiseParameters=[]  Unit=1  AffineConversion=off  FilteringAndDerivatives=zero  SimscapeFilterOrder=1  InputFilterTimeConstant=0.001  UdotUserProvided=1
  Sum : Sum  Inputs=-+|
  Switch : Switch  Criteria=u2 > Threshold
  Wheel and Axle : fl_lib/Mechanical/Mechanisms/Wheel and Axle  R=wheelRadius m  or=1  t_specify=off  t_priority=None  t=0 N*m  t_nominal_specify=off  t_nominal_unit=N*m  t_nominal_value=1  f_specify=off  f_priority=None  f=0 N  f_nominal_specify=off  f_nominal_unit=N  f_nominal_value=1
      settings: SourceProductName=Simscape
  Angular position : PMIOPort  Side=Right
  Position : PMIOPort  Port=2  Side=Right
  rpm : Outport
  P : Outport  Port=2
  wires:
  PS-Simulink Converter2/1 -> Gain1/1  "Ft"
  Gain1/1 -> rpm/1
  Fg/1 -> Simulink-PS Converter2/1
  PID Controller/1 -> Product1/2, Simulink-PS Converter1/1
  PS-Simulink Converter1/1 -> Gain2/1
  omega/1 -> Scope/3, Sum/2
  Gain2/1 -> Scope/2, Sum/1
  Encendido/1 -> Switch/2
  OFF/1 -> Switch/3
  Switch/1 -> PID Controller/1
  Sum/1 -> Switch/1
  PS-Simulink Converter3/1 -> Par/1
  PS-Simulink Converter4/1 -> Product1/1
  Product1/1 -> P/1
  connections:
  Inertia/LConn1 -- Rotational Friction/LConn1 -- Gear Box/RConn1 -- Ideal Rotational Motion Sensor/RConn1 -- Wheel and Axle/LConn1
  DC Motor/RConn2 -- Mechanical Rotational Reference/LConn1
  Ideal Rotational Motion Sensor1/LConn1 -- Ideal Torque Sensor/LConn1 -- DC Motor/LConn2
  Mechanical Translational Reference/LConn1 -- Ideal Translational Motion Sensor/RConn1
  Electrical Reference/LConn1 -- DC Motor/RConn1 -- Controlled Voltage Source/RConn2
  Simulink-PS Converter1/RConn1 -- Controlled Voltage Source/RConn1
  Mechanical Rotational Reference1/LConn1 -- Rotational Friction/RConn1
  Ideal Rotational Motion Sensor/RConn3 -- Angular position/RConn1
  Ideal Translational Motion Sensor/RConn3 -- Position/RConn1
  Mechanical Rotational Reference2/LConn1 -- Ideal Rotational Motion Sensor1/RConn1 -- Ideal Rotational Motion Sensor/LConn1
  Ideal Rotational Motion Sensor1/RConn2 -- PS-Simulink Converter2/LConn1
  Simulink-PS Converter2/RConn1 -- Ideal Force Source/RConn1
  Mechanical Translational Reference1/LConn1 -- Ideal Force Source/RConn2
  Ideal Translational Motion Sensor/LConn1 -- Wheel and Axle/RConn1 -- Ideal Force Source/LConn1 -- Mass/LConn1
  Ideal Rotational Motion Sensor/RConn2 -- PS-Simulink Converter1/LConn1
  Ideal Torque Sensor/RConn1 -- Gear Box/LConn1
  Ideal Torque Sensor/RConn2 -- PS-Simulink Converter3/LConn1
  Controlled Voltage Source/LConn1 -- Current Limiter/LConn1
  Current Sensor/RConn1 -- PS-Simulink Converter4/LConn1
  Current Limiter/RConn1 -- Current Sensor/LConn1
  Current Sensor/RConn2 -- DC Motor/LConn1

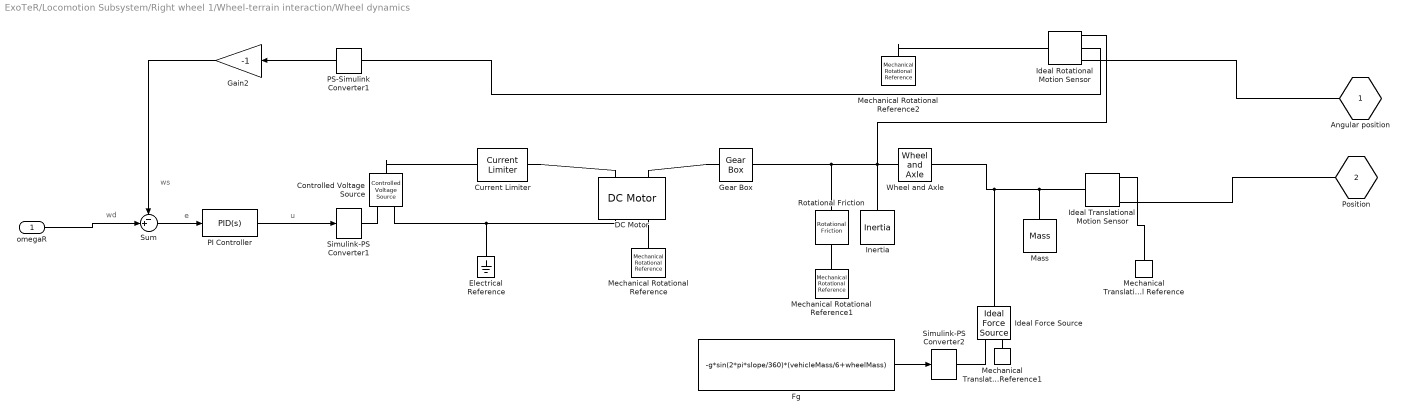
== system ExoTeR/Locomotion Subsystem/Right wheel 1/Wheel-terrain interaction/Wheel dynamics ==
  note: u
  note: e
  note: wd
  note: ws
  omegaR : Inport
  Controlled Voltage Source : fl_lib/Electrical/Electrical Sources/Controlled Voltage Source
  Current Limiter : ee_lib/Semiconductors & Converters/Current Limiter  iLim=0.5 A  vLim=0.01 V  gLim=1e-3 1/Ohm  thermal_mass=100 J/K  initial_temperature=298.15 K
      settings: SourceProductName=Simscape Electrical  SourceProductBaseCode=PS  InternalSimscapePortConfiguration="{\"Bottom\":[],\"Left\":[{\"id\":\"p\",\"label\":\"+\",\"type\":\"foundation.electrical.electrical\"}],\"Right\":[{\"id\":\"n\",\"label\":\"-\",\"type\":\"foundation.electrical.electrical\"}],\"Top\":[]}"
  DC Motor : ee_lib/Electromechanical/Brushed Motors/DC Motor  parameterization=2  Ra=3.9 Ohm  La=0.000363 H  emf_or_torque=2  Kv=0.0011 V/rpm  Ki=10.9 mN*m/A  T_stall=0.0237 N*m  w_max=10200 rpm  w_rated=1.5e+4 rpm  P_rated=0.08 W  V_rated=12 V  J=4.36 g*cm^2  lam_param=2  lam=Bm N*m/(rad/s)  i_noload=0.0458 A  V_i_noload=11.657 V  speed0=0 rpm  alpha=3.93e-3 1/K  Tmeas=25 degC  thermal_mass=100 J/K  initial_temperature=25 degC
      settings: SourceProductName=Simscape Electrical
  Electrical Reference : fl_lib/Electrical/Electrical Elements/Electrical Reference
  Fg : Constant  Value=-g*sin(2*pi*slope/360)*(vehicleMass/6+wheelMass)
  Gain2 : Gain  Gain=-1
  Gear Box : fl_lib/Mechanical/Mechanisms/Gear Box  ratio=675.545  t_in_specify=off  t_in_priority=None  t_in=0 N*m  t_in_nominal_specify=off  t_in_nominal_unit=N*m  t_in_nominal_value=1  t_out_specify=off  t_out_priority=None  t_out=0 N*m  t_out_nominal_specify=off  t_out_nominal_unit=N*m  t_out_nominal_value=1
  Ideal Force Source : fl_lib/Mechanical/Mechanical Sources/Ideal Force Source
  Ideal Rotational Motion Sensor : fl_lib/Mechanical/Mechanical Sensors/Ideal Rotational Motion Sensor  offset=0 rad
  Ideal Translational Motion Sensor : fl_lib/Mechanical/Mechanical Sensors/Ideal Translational Motion Sensor  offset=0 m
  Inertia : fl_lib/Mechanical/Rotational Elements/Inertia  inertia=Jw kg*m^2  w_specify=off  w_priority=None  w=0 rad/s  w_nominal_specify=off  w_nominal_unit=rad/s  w_nominal_value=1  t_specify=off  t_priority=None  t=0 N*m  t_nominal_specify=off  t_nominal_unit=N*m  t_nominal_value=1
  Mass : fl_lib/Mechanical/Translational Elements/Mass  mass=vehicleMass/6+wheelMass kg  v_specify=off  v_priority=None  v=0 m/s  v_nominal_specify=off  v_nominal_unit=m/s  v_nominal_value=1  f_specify=off  f_priority=None  f=0 N  f_nominal_specify=off  f_nominal_unit=N  f_nominal_value=1
  Mechanical Rotational Reference : fl_lib/Mechanical/Rotational Elements/Mechanical Rotational Reference
  Mechanical Rotational Reference1 : fl_lib/Mechanical/Rotational Elements/Mechanical Rotational Reference
  Mechanical Rotational Reference2 : fl_lib/Mechanical/Rotational Elements/Mechanical Rotational Reference
  Mechanical Translational Reference : fl_lib/Mechanical/Translational Elements/Mechanical Translational Reference
  Mechanical Translational Reference1 : fl_lib/Mechanical/Translational Elements/Mechanical Translational Reference
  PI Controller : simulink/Continuous/PID Controller  Controller=PID  Form=Parallel  TimeDomain=Continuous-time  SampleTime=-1  IntegratorMethod=Forward Euler  FilterMethod=Forward Euler  ControllerParametersSource=internal  P=kp  I=ki  D=0  UseFilter=on  N=100  TunerSelectOption=Transfer Function Based (PID Tuner App)  InitialConditionSource=internal  InitialConditionForIntegrator=0  InitialConditionForFilter=0  DifferentiatorICPrevScaledInput=0  ExternalReset=none  TrackingMode=off  Kt=1  LimitOutput=on  UpperSaturationLimit=12  LowerSaturationLimit=-12  LinearizeAsGain=on  AntiWindupMode=back-calculation  Kb=1  POutMin=[]  POutMax=[]  IOutMin=[]  IOutMax=[]  DOutMin=[]  DOutMax=[]  NOutMin=[]  NOutMax=[]  SumOutMin=[]  SumOutMax=[]  SaturationOutMin=[]  SaturationOutMax=[]  PParamMin=[]  PParamMax=[]  IParamMin=[]  IParamMax=[]  DParamMin=[]  DParamMax=[]  NParamMin=[]  NParamMax=[]  KbParamMin=[]  KbParamMax=[]  KtParamMin=[]  KtParamMax=[]  KbOutMin=[]  KbOutMax=[]  KtOutMin=[]  KtOutMax=[]  IntegratorOutMin=[]  IntegratorOutMax=[]  FilterOutMin=[]  FilterOutMax=[]  SumI1OutMin=[]  SumI1OutMax=[]  SumI2OutMin=[]  SumI2OutMax=[]  SumI3OutMin=[]  SumI3OutMax=[]  SumI4OutMin=[]  SumI4OutMax=[]  SumDOutMin=[]  SumDOutMax=[]  DifferentiatorOutMin=[]  DifferentiatorOutMax=[]  FilterDiffOutCoefMin=[]  FilterDiffOutCoefMax=[]  ReciprocalOutMin=[]  ReciprocalOutMax=[]  SumDenOutMin=[]  SumDenOutMax=[]  SumNumOutMin=[]  SumNumOutMax=[]  DivideOutMin=[]  DivideOutMax=[]  IntegratorContinuousStateAttributes=''  IntegratorStateMustResolveToSignalObject=off  IntegratorRTWStateStorageClass=Auto  FilterContinuousStateAttributes=''  FilterStateMustResolveToSignalObject=off  FilterRTWStateStorageClass=Auto  ParallelPVariant=InternalParameters  IdealPVariant=Disabled  IVariant=InternalParameters  DVariant=InternalParameters  IntegratorVariant=Continuous  SatVariant=Enabled  AWVariant=BackCalculation  PCopyVariant=Disabled  TRVariant=Disabled  FdbkBlocksVariant=Forward  IdealPFdbkVariant=Disabled  SatFdbkVariant=Disabled  DerivativeFilterVariant=ContFilter  NVariant=InternalParameters  NCopyVariant=Disabled  FilterICVariant=InternalICsFilter  IntegratorICVariant=InternalICs  ExternalResetVariant=Disabled  TRSumVariant=Passthrough  SumFdbkVariant=Disabled  SumVariant=Sum_PID
  PS-Simulink Converter1 : nesl_utility/PS-Simulink Converter  PhysicalDomain=network_engine_domain  SubClassName=ps_output  LeftPortType=input  RightPortType=output  PseudoPeriodic=off  Frequencies=[]  Unit=1  AffineConversion=off
  Rotational Friction : fl_lib/Mechanical/Rotational Elements/Rotational Friction  brkwy_trq=(vehicleMass/6+wheelMass)*g*cos(2*pi*slope/360)*mu*wheelRadius*s + (vehicleMass/6+wheelMass)*g*cos(2*pi*slope/360)*mu*0.1*wheelRadius*(1-s) N*m  brkwy_vel=0.060623 rad/s  Col_trq=((vehicleMass/6+wheelMass)*g*cos(2*pi*slope/360)*mu*wheelRadius*s + (vehicleMass/6+wheelMass)*g*cos(2*pi*slope/360)*mu*0.1*wheelRadius*(1-s))*0.9 N*m  visc_coef=0.001 N*m/(rad/s)  w_specify=off  w_priority=None  w=0 rad/s  w_nominal_specify=off  w_nominal_unit=rad/s  w_nominal_value=1  t_specify=off  t_priority=None  t=0 N*m  t_nominal_specify=off  t_nominal_unit=N*m  t_nominal_value=1
      settings: SourceProductName=Simscape
  Simulink-PS Converter1 : nesl_utility/Simulink-PS Converter  PhysicalDomain=network_engine_domain  SubClassName=ps_input  LeftPortType=input  RightPortType=output  PseudoPeriodic=off  Frequencies=[]  NoiseDistribution=none  NoiseParameters=[]  Unit=1  AffineConversion=off  FilteringAndDerivatives=zero  SimscapeFilterOrder=1  InputFilterTimeConstant=0.001  UdotUserProvided=1
  Simulink-PS Converter2 : nesl_utility/Simulink-PS Converter  PhysicalDomain=network_engine_domain  SubClassName=ps_input  LeftPortType=input  RightPortType=output  PseudoPeriodic=off  Frequencies=[]  NoiseDistribution=none  NoiseParameters=[]  Unit=1  AffineConversion=off  FilteringAndDerivatives=zero  SimscapeFilterOrder=1  InputFilterTimeConstant=0.001  UdotUserProvided=1
  Sum : Sum  Inputs=-+|
  Wheel and Axle : fl_lib/Mechanical/Mechanisms/Wheel and Axle  R=wheelRadius*(1-s) m  or=1  t_specify=off  t_priority=None  t=0 N*m  t_nominal_specify=off  t_nominal_unit=N*m  t_nominal_value=1  f_specify=off  f_priority=None  f=0 N  f_nominal_specify=off  f_nominal_unit=N  f_nominal_value=1
      settings: SourceProductName=Simscape
  Angular position : PMIOPort  Side=Right
  Position : PMIOPort  Port=2  Side=Right
  wires:
  Fg/1 -> Simulink-PS Converter2/1
  PI Controller/1 -> Simulink-PS Converter1/1
  PS-Simulink Converter1/1 -> Gain2/1
  omegaR/1 -> Sum/2
  Gain2/1 -> Sum/1
  Sum/1 -> PI Controller/1
  connections:
  Inertia/LConn1 -- Rotational Friction/LConn1 -- Gear Box/RConn1 -- Ideal Rotational Motion Sensor/RConn1 -- Wheel and Axle/LConn1
  DC Motor/RConn2 -- Mechanical Rotational Reference/LConn1
  Mechanical Translational Reference/LConn1 -- Ideal Translational Motion Sensor/RConn1
  Electrical Reference/LConn1 -- DC Motor/RConn1 -- Controlled Voltage Source/RConn2
  Simulink-PS Converter1/RConn1 -- Controlled Voltage Source/RConn1
  Rotational Friction/RConn1 -- Mechanical Rotational Reference1/LConn1
  Ideal Rotational Motion Sensor/RConn3 -- Angular position/RConn1
  Ideal Translational Motion Sensor/RConn3 -- Position/RConn1
  Mechanical Rotational Reference2/LConn1 -- Ideal Rotational Motion Sensor/LConn1
  Simulink-PS Converter2/RConn1 -- Ideal Force Source/RConn1
  Mechanical Translational Reference1/LConn1 -- Ideal Force Source/RConn2
  Ideal Translational Motion Sensor/LConn1 -- Wheel and Axle/RConn1 -- Ideal Force Source/LConn1 -- Mass/LConn1
  Ideal Rotational Motion Sensor/RConn2 -- PS-Simulink Converter1/LConn1
  Gear Box/LConn1 -- DC Motor/LConn2
  Controlled Voltage Source/LConn1 -- Current Limiter/LConn1
  Current Limiter/RConn1 -- DC Motor/LConn1

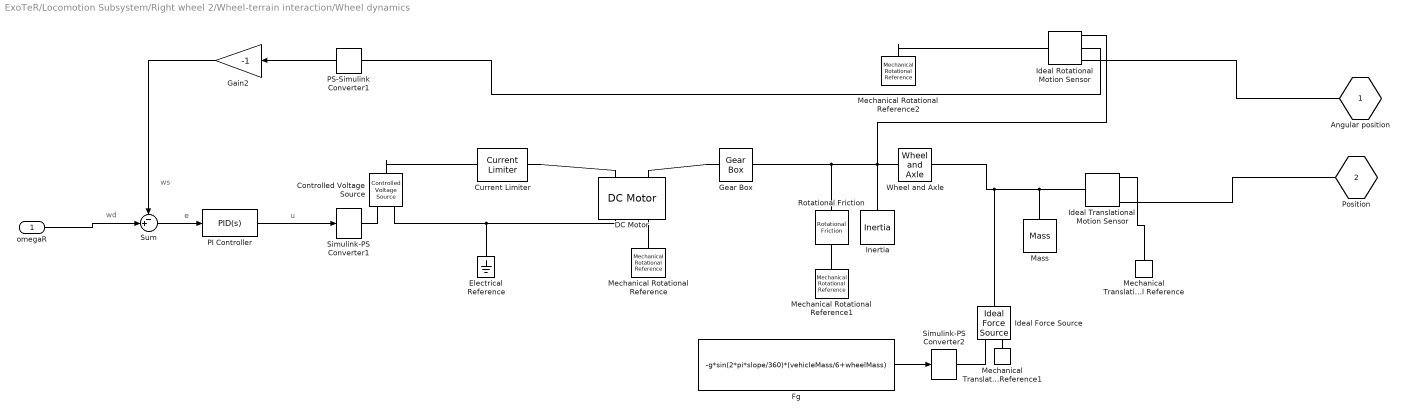
== system ExoTeR/Locomotion Subsystem/Right wheel 2/Wheel-terrain interaction/Wheel dynamics ==
  note: u
  note: e
  note: wd
  note: ws
  omegaR : Inport
  Controlled Voltage Source : fl_lib/Electrical/Electrical Sources/Controlled Voltage Source
  Current Limiter : ee_lib/Semiconductors & Converters/Current Limiter  iLim=0.5 A  vLim=0.01 V  gLim=1e-3 1/Ohm  thermal_mass=100 J/K  initial_temperature=298.15 K
      settings: SourceProductName=Simscape Electrical  SourceProductBaseCode=PS  InternalSimscapePortConfiguration="{\"Bottom\":[],\"Left\":[{\"id\":\"p\",\"label\":\"+\",\"type\":\"foundation.electrical.electrical\"}],\"Right\":[{\"id\":\"n\",\"label\":\"-\",\"type\":\"foundation.electrical.electrical\"}],\"Top\":[]}"
  DC Motor : ee_lib/Electromechanical/Brushed Motors/DC Motor  parameterization=2  Ra=3.9 Ohm  La=0.000363 H  emf_or_torque=2  Kv=0.0011 V/rpm  Ki=10.9 mN*m/A  T_stall=0.0237 N*m  w_max=10200 rpm  w_rated=1.5e+4 rpm  P_rated=0.08 W  V_rated=12 V  J=4.36 g*cm^2  lam_param=2  lam=Bm N*m/(rad/s)  i_noload=0.0458 A  V_i_noload=11.657 V  speed0=0 rpm  alpha=3.93e-3 1/K  Tmeas=25 degC  thermal_mass=100 J/K  initial_temperature=25 degC
      settings: SourceProductName=Simscape Electrical
  Electrical Reference : fl_lib/Electrical/Electrical Elements/Electrical Reference
  Fg : Constant  Value=-g*sin(2*pi*slope/360)*(vehicleMass/6+wheelMass)
  Gain2 : Gain  Gain=-1
  Gear Box : fl_lib/Mechanical/Mechanisms/Gear Box  ratio=675.545  t_in_specify=off  t_in_priority=None  t_in=0 N*m  t_in_nominal_specify=off  t_in_nominal_unit=N*m  t_in_nominal_value=1  t_out_specify=off  t_out_priority=None  t_out=0 N*m  t_out_nominal_specify=off  t_out_nominal_unit=N*m  t_out_nominal_value=1
  Ideal Force Source : fl_lib/Mechanical/Mechanical Sources/Ideal Force Source
  Ideal Rotational Motion Sensor : fl_lib/Mechanical/Mechanical Sensors/Ideal Rotational Motion Sensor  offset=0 rad
  Ideal Translational Motion Sensor : fl_lib/Mechanical/Mechanical Sensors/Ideal Translational Motion Sensor  offset=0 m
  Inertia : fl_lib/Mechanical/Rotational Elements/Inertia  inertia=Jw kg*m^2  w_specify=off  w_priority=None  w=0 rad/s  w_nominal_specify=off  w_nominal_unit=rad/s  w_nominal_value=1  t_specify=off  t_priority=None  t=0 N*m  t_nominal_specify=off  t_nominal_unit=N*m  t_nominal_value=1
  Mass : fl_lib/Mechanical/Translational Elements/Mass  mass=vehicleMass/6+wheelMass kg  v_specify=off  v_priority=None  v=0 m/s  v_nominal_specify=off  v_nominal_unit=m/s  v_nominal_value=1  f_specify=off  f_priority=None  f=0 N  f_nominal_specify=off  f_nominal_unit=N  f_nominal_value=1
  Mechanical Rotational Reference : fl_lib/Mechanical/Rotational Elements/Mechanical Rotational Reference
  Mechanical Rotational Reference1 : fl_lib/Mechanical/Rotational Elements/Mechanical Rotational Reference
  Mechanical Rotational Reference2 : fl_lib/Mechanical/Rotational Elements/Mechanical Rotational Reference
  Mechanical Translational Reference : fl_lib/Mechanical/Translational Elements/Mechanical Translational Reference
  Mechanical Translational Reference1 : fl_lib/Mechanical/Translational Elements/Mechanical Translational Reference
  PI Controller : simulink/Continuous/PID Controller  Controller=PID  Form=Parallel  TimeDomain=Continuous-time  SampleTime=-1  IntegratorMethod=Forward Euler  FilterMethod=Forward Euler  ControllerParametersSource=internal  P=kp  I=ki  D=0  UseFilter=on  N=100  TunerSelectOption=Transfer Function Based (PID Tuner App)  InitialConditionSource=internal  InitialConditionForIntegrator=0  InitialConditionForFilter=0  DifferentiatorICPrevScaledInput=0  ExternalReset=none  TrackingMode=off  Kt=1  LimitOutput=on  UpperSaturationLimit=12  LowerSaturationLimit=-12  LinearizeAsGain=on  AntiWindupMode=back-calculation  Kb=1  POutMin=[]  POutMax=[]  IOutMin=[]  IOutMax=[]  DOutMin=[]  DOutMax=[]  NOutMin=[]  NOutMax=[]  SumOutMin=[]  SumOutMax=[]  SaturationOutMin=[]  SaturationOutMax=[]  PParamMin=[]  PParamMax=[]  IParamMin=[]  IParamMax=[]  DParamMin=[]  DParamMax=[]  NParamMin=[]  NParamMax=[]  KbParamMin=[]  KbParamMax=[]  KtParamMin=[]  KtParamMax=[]  KbOutMin=[]  KbOutMax=[]  KtOutMin=[]  KtOutMax=[]  IntegratorOutMin=[]  IntegratorOutMax=[]  FilterOutMin=[]  FilterOutMax=[]  SumI1OutMin=[]  SumI1OutMax=[]  SumI2OutMin=[]  SumI2OutMax=[]  SumI3OutMin=[]  SumI3OutMax=[]  SumI4OutMin=[]  SumI4OutMax=[]  SumDOutMin=[]  SumDOutMax=[]  DifferentiatorOutMin=[]  DifferentiatorOutMax=[]  FilterDiffOutCoefMin=[]  FilterDiffOutCoefMax=[]  ReciprocalOutMin=[]  ReciprocalOutMax=[]  SumDenOutMin=[]  SumDenOutMax=[]  SumNumOutMin=[]  SumNumOutMax=[]  DivideOutMin=[]  DivideOutMax=[]  IntegratorContinuousStateAttributes=''  IntegratorStateMustResolveToSignalObject=off  IntegratorRTWStateStorageClass=Auto  FilterContinuousStateAttributes=''  FilterStateMustResolveToSignalObject=off  FilterRTWStateStorageClass=Auto  ParallelPVariant=InternalParameters  IdealPVariant=Disabled  IVariant=InternalParameters  DVariant=InternalParameters  IntegratorVariant=Continuous  SatVariant=Enabled  AWVariant=BackCalculation  PCopyVariant=Disabled  TRVariant=Disabled  FdbkBlocksVariant=Forward  IdealPFdbkVariant=Disabled  SatFdbkVariant=Disabled  DerivativeFilterVariant=ContFilter  NVariant=InternalParameters  NCopyVariant=Disabled  FilterICVariant=InternalICsFilter  IntegratorICVariant=InternalICs  ExternalResetVariant=Disabled  TRSumVariant=Passthrough  SumFdbkVariant=Disabled  SumVariant=Sum_PID
  PS-Simulink Converter1 : nesl_utility/PS-Simulink Converter  PhysicalDomain=network_engine_domain  SubClassName=ps_output  LeftPortType=input  RightPortType=output  PseudoPeriodic=off  Frequencies=[]  Unit=1  AffineConversion=off
  Rotational Friction : fl_lib/Mechanical/Rotational Elements/Rotational Friction  brkwy_trq=(vehicleMass/6+wheelMass)*g*cos(2*pi*slope/360)*mu*wheelRadius*s + (vehicleMass/6+wheelMass)*g*cos(2*pi*slope/360)*mu*0.1*wheelRadius*(1-s) N*m  brkwy_vel=0.060623 rad/s  Col_trq=((vehicleMass/6+wheelMass)*g*cos(2*pi*slope/360)*mu*wheelRadius*s + (vehicleMass/6+wheelMass)*g*cos(2*pi*slope/360)*mu*0.1*wheelRadius*(1-s))*0.9 N*m  visc_coef=0.001 N*m/(rad/s)  w_specify=off  w_priority=None  w=0 rad/s  w_nominal_specify=off  w_nominal_unit=rad/s  w_nominal_value=1  t_specify=off  t_priority=None  t=0 N*m  t_nominal_specify=off  t_nominal_unit=N*m  t_nominal_value=1
      settings: SourceProductName=Simscape
  Simulink-PS Converter1 : nesl_utility/Simulink-PS Converter  PhysicalDomain=network_engine_domain  SubClassName=ps_input  LeftPortType=input  RightPortType=output  PseudoPeriodic=off  Frequencies=[]  NoiseDistribution=none  NoiseParameters=[]  Unit=1  AffineConversion=off  FilteringAndDerivatives=zero  SimscapeFilterOrder=1  InputFilterTimeConstant=0.001  UdotUserProvided=1
  Simulink-PS Converter2 : nesl_utility/Simulink-PS Converter  PhysicalDomain=network_engine_domain  SubClassName=ps_input  LeftPortType=input  RightPortType=output  PseudoPeriodic=off  Frequencies=[]  NoiseDistribution=none  NoiseParameters=[]  Unit=1  AffineConversion=off  FilteringAndDerivatives=zero  SimscapeFilterOrder=1  InputFilterTimeConstant=0.001  UdotUserProvided=1
  Sum : Sum  Inputs=-+|
  Wheel and Axle : fl_lib/Mechanical/Mechanisms/Wheel and Axle  R=wheelRadius*(1-s) m  or=1  t_specify=off  t_priority=None  t=0 N*m  t_nominal_specify=off  t_nominal_unit=N*m  t_nominal_value=1  f_specify=off  f_priority=None  f=0 N  f_nominal_specify=off  f_nominal_unit=N  f_nominal_value=1
      settings: SourceProductName=Simscape
  Angular position : PMIOPort  Side=Right
  Position : PMIOPort  Port=2  Side=Right
  wires:
  Fg/1 -> Simulink-PS Converter2/1
  PI Controller/1 -> Simulink-PS Converter1/1
  PS-Simulink Converter1/1 -> Gain2/1
  omegaR/1 -> Sum/2
  Gain2/1 -> Sum/1
  Sum/1 -> PI Controller/1
  connections:
  Inertia/LConn1 -- Rotational Friction/LConn1 -- Gear Box/RConn1 -- Ideal Rotational Motion Sensor/RConn1 -- Wheel and Axle/LConn1
  DC Motor/RConn2 -- Mechanical Rotational Reference/LConn1
  Mechanical Translational Reference/LConn1 -- Ideal Translational Motion Sensor/RConn1
  Electrical Reference/LConn1 -- DC Motor/RConn1 -- Controlled Voltage Source/RConn2
  Simulink-PS Converter1/RConn1 -- Controlled Voltage Source/RConn1
  Rotational Friction/RConn1 -- Mechanical Rotational Reference1/LConn1
  Ideal Rotational Motion Sensor/RConn3 -- Angular position/RConn1
  Ideal Translational Motion Sensor/RConn3 -- Position/RConn1
  Mechanical Rotational Reference2/LConn1 -- Ideal Rotational Motion Sensor/LConn1
  Simulink-PS Converter2/RConn1 -- Ideal Force Source/RConn1
  Mechanical Translational Reference1/LConn1 -- Ideal Force Source/RConn2
  Ideal Translational Motion Sensor/LConn1 -- Wheel and Axle/RConn1 -- Ideal Force Source/LConn1 -- Mass/LConn1
  Ideal Rotational Motion Sensor/RConn2 -- PS-Simulink Converter1/LConn1
  Gear Box/LConn1 -- DC Motor/LConn2
  Controlled Voltage Source/LConn1 -- Current Limiter/LConn1
  Current Limiter/RConn1 -- DC Motor/LConn1
